simulink model "da5_control"  (R2017b)
settings: Solver=VariableStepAuto  StartTime=0.0  StopTime=5  RelTol=1e-9
settings Model: Creator=chenjiasheng  LastModifiedBy=chenjiasheng

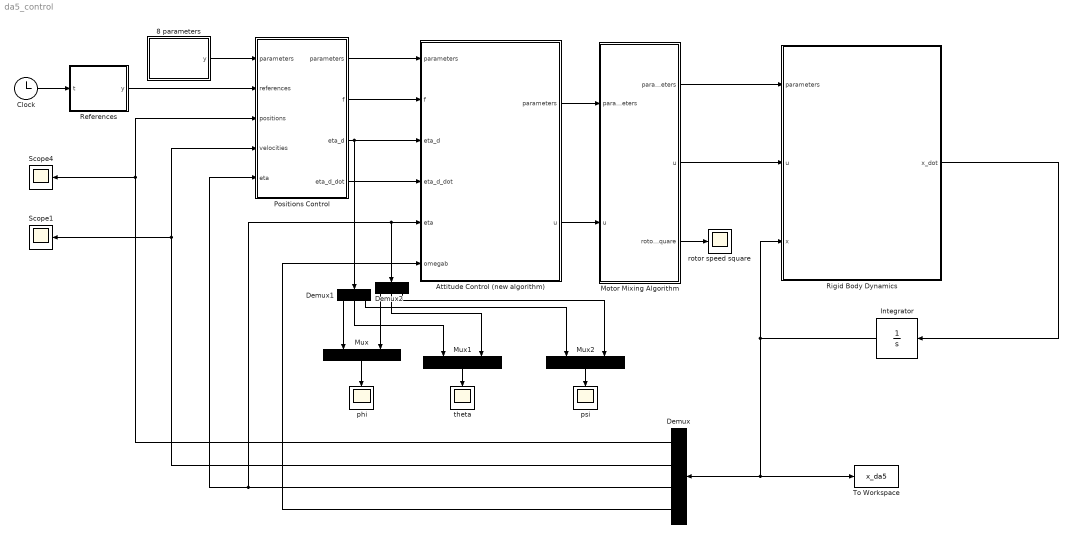
== system da5_control ==
  8 parameters : MATLAB Function  TreatAsAtomicUnit=on
  Attitude Control (new algorithm) : MATLAB Function  TreatAsAtomicUnit=on
  Clock : Clock
  Demux : Demux
  Demux1 : Demux  Outputs=3
  Demux2 : Demux  Outputs=3
  Integrator : Integrator  InitialCondition=x_da4(end,:)  ContinuousStateAttributes='x'
  Motor Mixing Algorithm : MATLAB Function  TreatAsAtomicUnit=on
  Mux : Mux  Inputs=2
  Mux1 : Mux  Inputs=2
  Mux2 : Mux  Inputs=2
  Positions Control : MATLAB Function  TreatAsAtomicUnit=on
  References : MATLAB Function  TreatAsAtomicUnit=on
  Rigid Body Dynamics : MATLAB Function  TreatAsAtomicUnit=on
  Scope1 : Scope
  Scope4 : Scope
  To Workspace : ToWorkspace  VariableName=x_da5  SampleTime=0.01
  phi : Scope
  psi : Scope
  rotor speed square : Scope
  theta : Scope
  wires:
  Motor Mixing Algorithm/1(parameters) -> Rigid Body Dynamics/1(parameters)
  Demux2/3 -> Mux2/2
  Motor Mixing Algorithm/3(rotor_speed_square) -> rotor speed square/1
  Mux/1 -> phi/1
  Clock/1 -> References/1(t)
  Demux/3 -> Positions Control/5(eta), Attitude Control (new algorithm)/5(eta), Demux2/1
  Demux/4 -> Attitude Control (new algorithm)/6(omegab)
  Demux2/1 -> Mux/2
  Motor Mixing Algorithm/2(u) -> Rigid Body Dynamics/2(u)
  Demux1/3 -> Mux2/1
  Demux/1 -> Scope4/1, Positions Control/3(positions)
  Demux1/2 -> Mux1/1
  Rigid Body Dynamics/1(x_dot) -> Integrator/1
  Mux2/1 -> psi/1
  References/1(y) -> Positions Control/2(references)
  Integrator/1 -> To Workspace/1, Demux/1, Rigid Body Dynamics/3(x)
  Positions Control/3(eta_d) -> Attitude Control (new algorithm)/3(eta_d), Demux1/1
  Demux2/2 -> Mux1/2
  Attitude Control (new algorithm)/1(parameters) -> Motor Mixing Algorithm/1("parameters ")
  Positions Control/2(f) -> Attitude Control (new algorithm)/2(f)
  Mux1/1 -> theta/1
  Attitude Control (new algorithm)/2(u) -> Motor Mixing Algorithm/2("u ")
  Positions Control/1(parameters) -> Attitude Control (new algorithm)/1("parameters ")
  8 parameters/1(y) -> Positions Control/1("parameters ")
  Positions Control/4(eta_d_dot) -> Attitude Control (new algorithm)/4(eta_d_dot)
  Demux1/1 -> Mux/1
  Demux/2 -> Positions Control/4(velocities), Scope1/1

== matlab function da5_control/Positions Control ==
  data: parameters input size=8; parameters output size=8; references input size=11; positions input size=3; velocities input size=3; f output size=1; eta_d output size=3; eta_d_dot output size=3; eta input size=3
 function [parameters,f,eta_d,eta_d_dot] =fcn(parameters,references,positions,velocities,eta)
%% kp,kd for the positions controller
kp=diag([10 10 10]); % kp=diag([kpx kpy kpz])
kd=diag([5 5 5]);    % kd=diag([kdx kdy kdz])
%% allocate inputs
m=parameters(1);
g=parameters(2);
r_d=references(1:3);  % reference's positions
r_d_dot=references(4:6);  % reference's velocities
r_d_dot_dot=references(7:9); % reference's accelerations
psi_d=references(10);    % reference's yaw angle 
psi_d_dot=references(11); % reference's yaw angle velocity
r=positions ;         % positions 
r_dot=velocities ;    % velocities
phi=eta(1);
theta=eta(2);
psi=eta(3);
Rbn=[cos(theta)*cos(psi) sin(phi)*sin(theta)*cos(psi)-cos(phi)*sin(psi) cos(phi)*sin(theta)*cos(psi)+sin(phi)*sin(psi);
     cos(theta)*sin(psi) sin(phi)*sin(theta)*sin(psi)+cos(phi)*cos(psi) cos(phi)*sin(theta)*sin(psi)-sin(phi)*cos(psi);
     -sin(theta)         sin(phi)*cos(theta)                            cos(phi)*cos(theta)                           ];

%% desired accelerations and jerk applied on the drone
a_d=kp*(r_d-r)+kd*(r_d_dot-r_dot);
f=m*sqrt(a_d(1)^2+a_d(2)^2+(g+a_d(3))^2);
r_dot_dot=1/m*Rbn*[0 0 f]'-[0 0 g]';
a_d_dot=kp*(r_d_dot-r_dot)+kd*(r_d_dot_dot-r_dot_dot) ;
% Note a_d and r_d_dot_dot are 2 different variables!
% a_d is the desired acceleration that is applied on the drone. a_d is derived from PD control law.
% r_d_dot_dot is the reference's accelerations, which was given already at the beginning. 
%% desired roll and pitch angle 
A=a_d(1)*sin(psi_d)-a_d(2)*cos(psi_d);
C=a_d(1)*cos(psi_d)+a_d(2)*sin(psi_d);
D=g+a_d(3);
B=sqrt(C^2+D^2);
phi_d=asin(A*m/f) ;
if C>0
theta_d=acos(D/B);
else
theta_d=-acos(D/B) ;
end
%% change rate of desired roll and pitch angles
phi_d_dot=(sin(psi_d)*(f/m)^2-A*a_d(1))/((f/m)^2*B)*a_d_dot(1) + (-cos(psi_d)*(f/m)^2-A*a_d(2))/((f/m)^2*B)*a_d_dot(2) + (-A*D)/((f/m)^2*B)*a_d_dot(3) + C/B*psi_d_dot ;
theta_d_dot=(cos(psi_d)*D*a_d_dot(1)+sin(psi_d)*D*a_d_dot(2)-C*a_d_dot(3)-A*D*psi_d_dot)/B^2  ;                                                                                                           
%% output                         
                                 %  1-8: eight parameters  
                                %  9: f
eta_d=[phi_d;theta_d;psi_d]    ;          %  10-12
eta_d_dot=[phi_d_dot;theta_d_dot;psi_d_dot] ;  %  13-15

== matlab function da5_control/8 parameters ==
  data: y output size=8
function y=fcn
%% specify parameters
m=3;
g=9.81;
Ix=4.856*10^(-3);
Iy=4.856*10^(-3);
Iz=8.801*10^(-3);
l=0.225;
k=2.980*10^-6;
c=1.140*10^-7;
%% output
y=[m;g;Ix;Iy;Iz;l;k;c] ;% output # 1-8
    
end

== matlab function da5_control/Attitude Control (new algorithm) ==
  data: parameters input size=8; parameters output size=8; f input size=1; eta_d input size=3; eta_d_dot input size=3; eta input size=3; omegab input size=3; u output size=4
function [parameters,u]=fcn(parameters,f,eta_d,eta_d_dot,eta,omegab)
%% kp, kd for the attitude control
kp=diag([150 150 150]); % kp_phi, kp_theta, kp_psi
kd=diag([22 22 22]); % kd_phi, kd_theta, kd_psi
%% allocate inputs
M=diag([parameters(3), parameters(4), parameters(5)]);
phi=eta(1);
theta=eta(2);
psi=eta(3);
eta_dot=[1 sin(phi)*tan(theta) cos(phi)*tan(theta);
         0 cos(phi)            -sin(phi);
         0 sin(phi)/cos(theta) cos(phi)/cos(theta)]*omegab;
phi_dot=eta_dot(1);
theta_dot=eta_dot(2);
psi_dot=eta_dot(3);
%% get taub
eta_dot_dot=kp*(eta_d-eta)+kd*(eta_d_dot-eta_dot);
phi_dot_dot=eta_dot_dot(1);
theta_dot_dot=eta_dot_dot(2);
psi_dot_dot=eta_dot_dot(3);
p_dot=phi_dot_dot-psi_dot_dot*sin(theta)-theta_dot*psi_dot*cos(theta) ;
q_dot=theta_dot_dot*cos(phi)+psi_dot_dot*sin(phi)*cos(theta)-phi_dot*theta_dot*sin(phi)+phi_dot*psi_dot*cos(phi)*cos(theta)-theta_dot*psi_dot*sin(phi)*sin(theta) ;
r_dot=-theta_dot_dot*sin(phi)+psi_dot_dot*cos(phi)*cos(theta)-phi_dot*theta_dot*cos(phi)-phi_dot*psi_dot*sin(phi)*cos(theta)-theta_dot*psi_dot*cos(phi)*sin(theta) ;
omegab_dot=[p_dot q_dot r_dot]' ;
taub=M*omegab_dot+cross(omegab,M*omegab) ;
%% u
u=[f;taub];

end

== matlab function da5_control/References ==
  data: t input; y output
function y = fcn(t)
%% specify your references here
r_desired=[4.2831 0 0]';  % reference's positions
r_desired_dot=[0 0 0]'; % reference's velocities
r_desired_dot_dot=[0 0 0]'; % reference's accelerations
psi_desired=0 ;      % reference's yaw angle
psi_desired_dot=0 ;  % reference's change rate of yaw angle                      
y=[ r_desired;           %  1-3
    r_desired_dot;       %  4-6
    r_desired_dot_dot;   %  7-9
    psi_desired;         %  10
    psi_desired_dot];    %  11

== matlab function da5_control/Motor Mixing Algorithm ==
  data: parameters output; u output; parameters input size=8; u input size=4; rotor_speed_square output size=4
function [parameters,u,rotor_speed_square]=fcn(parameters,u)
l=parameters(6) ; 
k=parameters(7) ;
c=parameters(8) ;
rotor_speed_square=[1 0 -1  1;
                    1 1  0 -1;
                    1 0  1  1;
                    1 -1 0 -1]* [1/(4*k) 0         0         0;
                                0        1/(2*l*k) 0         0;
                                0        0         1/(2*l*k) 0;
                                0        0         0         1/(4*c)]*u ;
end
%% Motor dynamics
% rotor_speed=in(9:12)
% rotor_speed_square=rotor_speed.^2
%f_taux_tauy_tauz=[k 0   0   0;
%                  0 k*l 0   0;
%                  0 0   k*l 0;
%                  0 0   0   c]*[1  1 1  1;
%                                0  1 0 -1;
%                               -1  0 1  0;
%                                1 -1 1 -1]*rotor_speed_square

== matlab function da5_control/Rigid Body Dynamics ==
  data: parameters input size=8; x_dot output size=12; u input size=4; x input size=12
function x_dot=fcn(parameters,u,x)
%% allocate inputs
m=parameters(1);
g=parameters(2);
M=diag([parameters(3) parameters(4) parameters(5)]);
f=u(1);
taub=u(2:4);
pn=x(1:3);
vn=x(4:6);
eta=x(7:9);
omegab=x(10:12);
%% define matrix Rbn , Lbn and Omega
phi=eta(1);
theta=eta(2);
psi=eta(3);
Rbn=[cos(theta)*cos(psi) sin(phi)*sin(theta)*cos(psi)-cos(phi)*sin(psi) cos(phi)*sin(theta)*cos(psi)+sin(phi)*sin(psi);
     cos(theta)*sin(psi) sin(phi)*sin(theta)*sin(psi)+cos(phi)*cos(psi) cos(phi)*sin(theta)*sin(psi)-sin(phi)*cos(psi);
     -sin(theta)         sin(phi)*cos(theta)                            cos(phi)*cos(theta)                           ];
Lbn=[1 sin(phi)*tan(theta) cos(phi)*tan(theta);
     0 cos(phi)            -sin(phi);
     0 sin(phi)/cos(theta) cos(phi)/cos(theta)];

%% nonlinear model: shown on the handout
pn_dot=vn;
vn_dot=1/m*Rbn*[0 0 f]'-[0 0 g]'; % -1/m*[Ax 0 0;0 Ay 0;0 0 Az]*pn_dot;    % pay attention to whether I need Ax, Ay, Az
eta_dot=Lbn*omegab;
omegab_dot=M\(taub-cross(omegab,M*omegab));
%% output x_dot
x_dot=[pn_dot;
       vn_dot;
       eta_dot;
       omegab_dot];
end
